simulink model "admire_sim_NDI"  (Simulink 9.1)
settings: Solver=ode4  StartTime=0.0  StopTime=500  FixedStep=dt  RelTol=1e-3  AbsTol=1e-6
InitFcn:
  | INIT_NDI
StartFcn:
  | tic
StopFcn:
  | toctime=toc;
  | fprintf('Actual Time = %g\nSim Time = %g\n',toctime,tout(end))
  | % Make plots
  | %admire_sim_plot
  | figure
  | plot3(yout(:,11),yout(:,10),-yout(:,12),'*-');grid
  | xlabel('East (m)');ylabel('North (m)');zlabel('Alt (m)')
  | view([0 0 1])
  | hold on
  | plot3(Ywpt,Xwpt,0*Xwpt,'r^-','MarkerSize',10)
  | axis equal
  | hold off
values from neighbouring files (symbols this model uses):
  a1 = (180*d2r)/(80^3)    (= 6.13592315154e-06)    [INIT_NDI.m]
  a2 = (24*d2r)/(80^3)    (= 8.18123086872e-07)    [INIT_NDI.m]
  Altcmd_t = [ 0    1   100 200  300  425  450  550  600  700  800  880  980]    [INIT_NDI.m]
  Altcmd_v = [20  20   20   1500 1500 1500 1500 3000 3000 4000 4000 6000 6000]    [INIT_NDI.m]
  bref = 10    [INIT_NDI.m]
  C1 = ((Iy-Iz)*Iz-Ixz^2)/GG    (= -0.958151081688)    [INIT_NDI.m]
  C2 = (Ix-Iy+Iz)*Ixz/GG    (= 0.0484690861804)    [INIT_NDI.m]
  C3 = Iz/GG    (= 4.77597824802e-05)    [INIT_NDI.m]
  C4 = Ixz/GG    (= 1.18217283367e-06)    [INIT_NDI.m]
  C5 = (Iz-Ix)/Iy    (= 0.987654320988)    [INIT_NDI.m]
  C6 = Ixz/Iy    (= 0.0308641975309)    [INIT_NDI.m]
  C7 = 1/Iy    (= 1.23456790123e-05)    [INIT_NDI.m]
  C8 = (Ix*(Ix-Iy)+Ixz^2)/GG    (= -0.592859676085)    [INIT_NDI.m]
  C9 = Ix/GG    (= 9.93025180281e-06)    [INIT_NDI.m]
  CAmethod = 6    [INIT_NDI.m]
  Canard_max = [25 25 25 15 15 15 15 15]*d2r    [INIT_NDI.m]
  Canard_min = [-55 -55 -25 -15 -15 -15 -15 -15]*d2r    [INIT_NDI.m]
  CB = CCV*Bbare    [INIT_NDI.m]
  CC = [C3 0 C4;0 C7 0;C4 0 C9]    [INIT_NDI.m]
  CCV = [CCV zeros(3,22)]    [INIT_NDI.m]
  cref = 5.2    [INIT_NDI.m]
  d2r = pi/180    (= 0.0174532925199)    [INIT_NDI.m]
  dt = 0.01    [INIT_NDI.m]
  DTY_max = 0.002    [INIT_NDI.m]
  DTY_min = -0.002    [INIT_NDI.m]
  DTZ_max = 0.002    [INIT_NDI.m]
  DTZ_min = -0.002    [INIT_NDI.m]
  du = [eye(7,7)*d2r eye(7,7)*(-d2r);zeros(20,14)]    [INIT_NDI.m]
  Elevon_max = [30 30 25 25 25 25 25 25]*d2r    [INIT_NDI.m]
  Elevon_min = [-30 -30 -30 -30 -30 -30 -30 -30]*d2r    [INIT_NDI.m]
  G = [ 0 1 0 ... (first row only)    [INIT_NDI.m]
  kcb = 2.5    [INIT_NDI.m]
  kfb = -0.4    [INIT_NDI.m]
  kib = 0.2    [INIT_NDI.m]
  kpb = 0.8    [INIT_NDI.m]
  LEF_max = [30 30 30 20 20 15 10 10]*d2r    [INIT_NDI.m]
  LEF_min = [-10 -10 -10 -10 -10 -10 -10 -10]*d2r    [INIT_NDI.m]
  LG_max = 1    [INIT_NDI.m]
  LG_min = 0    [INIT_NDI.m]
  LPmethod = 5    [INIT_NDI.m]    (also in LPwrap.m = 0)
  M_vec = [0 0.5 0.8 0.9 0.95 1.4 1.5 2.5]    [INIT_NDI.m]
  mass = 9100    [INIT_NDI.m]
  NumU = 16    [INIT_NDI.m]
  nwpt = 5    [INIT_NDI.m]
  PD_max = 10    [INIT_NDI.m]
  PD_min = -10    [INIT_NDI.m]
  PHIcmd_t = [0 1 1+dt 30 30+dt 60 60+dt 90 90+dt 120 120+dt 150 150+dt 180 180+dt 210 210+dt 240 240+dt 270 270+dt 300 300+dt 330 330+dt]    [INIT_NDI.m]
  PHIcmd_v = [0 0 15   15 -15   -15 0    0   30   30  -30    -30 0      0   45     45   0     0    -45   -45   0     0   -60   -60 0]    [INIT_NDI.m]
  Pmode = 3    [INIT_NDI.m]
  r2d = 180/pi    (= 57.2957795131)    [INIT_NDI.m]
  Rmode = 3    [INIT_NDI.m]
  Rudder_max = [30 30 25 20 15 15 15 10]*d2r    [INIT_NDI.m]
  Rudder_min = [-30 -30 -25 -20 -15 -15 -15 -10]*d2r    [INIT_NDI.m]
  Sref = 45    [INIT_NDI.m]
  TSS_max = 1    [INIT_NDI.m]
  TSS_min = 0    [INIT_NDI.m]
  UD_max = 10    [INIT_NDI.m]
  UD_min = -10    [INIT_NDI.m]
  Upref = [0 0 0 0 0 0 0 0 0 0 0 0 0 0 0 0]'    [INIT_NDI.m]
  Upref_split = [[0 0 30 -30 -30 30 0]*d2r*.4 0 0 0 0 0 0 0 0 0]'    [INIT_NDI.m]
  Urlim = [50*d2r ... (first row only)    [INIT_NDI.m]
  UseRL = 0    [INIT_NDI.m]
  Vcmd_t = [  0    1   100  200  300  425  450  550  600  700  800  880  980]    [INIT_NDI.m]
  Vcmd_v = Mcmd_v.*a    [INIT_NDI.m]
  VD_max = 10    [INIT_NDI.m]
  VD_min = -10    [INIT_NDI.m]
  WD_max = 10    [INIT_NDI.m]
  WD_min = -10    [INIT_NDI.m]
  Wp = W'*W    [INIT_NDI.m]
  Wpts = [0 1 2 3 4]    [INIT_NDI.m]
  x0 = [ max(eyp,zeros(n,1));max(-eyp,zeros(n,1));zeros(2*m,1)]    [LPwrap.m]
  Xwpt = [0 4000 4000 0 0]*8    [INIT_NDI.m]
  Ywpt = [0 0 4000 4000 0]*8    [INIT_NDI.m]
undefined symbols (not defined in the file or in its folder): Abare, Bbare, CGIwrap, dalpha_err, dalt_err, DAwrap, dbeta_err, ddc_bw, ddc_rate, ddei_bw, ddei_rate, ddey_bw, ddey_rate, ddle_bw, ddle_rate, ddr_bw, ddr_rate, DiscIntNeverNeededParam, dVt_err, LPwrap, rlimit_c, rlimit_ie, rlimit_le, rlimit_oe, rlimit_r, u0fcs, u0new, VJAwrap, x0bare, y0bare
libraries: simulink_extras x19, simulink x12
(part 1 of 4)
settings Model: Creator=ulrik  LastModifiedBy=Meng Chaoheng  ModifiedComment=nnt -- Mon Jun 05 13:08:11 2000 -- Version 3.42  ExtModeTrigMode=oneshot  ExtModeArmWhenConnect=off  ExtModeAutoUpdateStatusClock=off
settings Model: ModifiedHistory=|
  | nnt -- Mon Jun 05 13:08:11 2000 -- Version 3.42
  | 
  | 
  | nnt -- Mon Jun 05 11:01:33 2000 -- Version 3.41
  | 
  | 
  | nnt -- Mon Jun 05 10:57:40 2000 -- Version 3.40
  | 
  | 
  | nnt -- Mon Jun 05 10:56:46 2000 -- Version 3.39
  | 
  | 
  | hkg -- Thu Apr 13 16:38:30 2000 -- Version 3.38
  | Bug fix: all rate limiters were set with the canard parameters, now they get individual settings..
  | 
  | hkg -- Thu Apr 13 10:24:31 2000 -- Version 3.37
  | Inserted 3.0 version number in Level 1, changed month to April.
  | 
  | hkg -- Tue Apr 11 10:36:55 2000 -- Version 3.36
  | dtz re-connected
  | 
  | hkg -- Tue Apr 11 10:28:52 2000 -- Version 3.35
  | Changed the roll force saturation to +-80 N
  | 
  | hkg -- Tue Apr 11 09:23:02 2000 -- Version 3.34
  | All signal generators on Level 1 are now set to sine wave
  | 
  | hkg -- Mon Apr 10 15:03:16 2000 -- Version 3.33
  | New names for the RL_choice blocks
  | 
  | fosimadmin -- Mon Apr 10 13:44:14 2000 -- Version 3.32
  | Hkg actually. Nothing special
  | 
  | hkg -- Fri Apr 07 14:32:16 2000 -- Version 3.31
  | A few corrections to the names
  | 
  | hkg -- Fri Apr 07 14:16:55 2000 -- Version 3.30
  | Added unique names inside Saab and DASA rate limiters for left elevons, rudder and
  | leading-edge flaps.
  | hkg -- Fri Apr 07 14:04:35 2000 -- Version 3.29
  | Added unique names inside SAAB and DASA rate limiters for canard and right outer and
  | inner elevons.
  | hkg -- Thu Apr 06 17:23:24 2000 -- Version 3.28
  | Inserted unique names for rate limiters and multiport switches in the rate limiter selection blocks.
  | hkg -- Thu Apr 06 16:09:22 2000 -- Version 3.27
  | Disconnected dtz again. Chosen grt_adm5p3.tmf as template makefile. Code generation seems to work.
  | hyd -- Tue Mar 28 15:20:39 2000 -- Version 3.26
  | hyd -- Tue Mar 28 14:28:32 2000 -- Version 3.25
  | hyd -- Tue Mar 28 11:30:24 2000 -- Version 3.24
  | hyd -- Mon Mar 27 15:22:27 2000 -- Version 3.23
  | hyd -- Mon Mar 27 13:42:12 2000 -- Version 3.22
  | hyd -- Mon Mar 27 10:51:54 2000 -- Version 3.21
  | hyd -- Fri Mar 24 13:18:05 2000 -- Version 3.20
  | hyd -- Fri Mar 24 12:50:02 2000 -- Version 3.19
  | hyd -- Fri Mar 24 11:54:23 2000 -- Version 3.18
  | hyd -- Thu Mar 23 15:20:42 2000 -- Version 3.17
  | hyd -- Thu Mar 23 15:17:54 2000 -- Version 3.16
  | hyd -- Wed Mar 22 09:38:49 2000 -- Version 3.15
  | hyd -- Tue Mar 21 14:06:08 2000 -- Version 3.14
  | hyd -- Mon Mar 20 14:42:54 2000 -- Version 3.13
  | hyd -- Wed Mar 15 13:37:48 2000 -- Version 3.12
  | hyd -- Wed Mar 15 12:35:54 2000 -- Version 3.11
  | jnr -- Tue Mar 14 16:36:26 2000 -- Version 3.10
  | jnr -- Tue Mar 14 14:13:39 2000 -- Version 3.9
  | jnr -- Tue Mar 14 14:13:23 2000 -- Version 3.8
  | jnr -- Tue Mar 14 10:09:15 2000 -- Version 3.7
  | jnr -- Tue Mar 14 09:37:34 2000 -- Version 3.6
  | jnr -- Tue Mar 14 09:30:20 2000 -- Version 3.5
  | Add:
  | *proper stick gradients.
  | *correct gains for nz-control according to ke Hydn.
  | *what transition region between q-control and nz-control is proper??
  | fll -- Fri Mar 03 09:53:48 2000 -- Version 3.4
  | changed name of "dtx" to "dty" (horizontal nozzle deflection)
  | fll -- Thu Mar 02 12:51:23 2000 -- Version 3.3
  | Reducesed the number of integrators to one in the longitudinal controller.
  | fll -- Thu Mar 02 12:30:52 2000 -- Version 3.2
  | Moved the blending function in the Nz and q controller.
  | fll -- Thu Mar 02 10:50:25 2000 -- Version 3.1
  | Changed input blocks to "Signal generator"
  | fll -- Thu Mar 02 10:50:25 2000 -- Version 3.0
  | Version 3.0 is modified according to comments from users
settings SolverCC: AutoScaleAbsTol=off
settings DataIOCC: SignalLoggingName=sigsOut
settings OptimizationCC: BooleanDataType=off  ExpressionDepthLimit=2147483647
settings DebuggingCC: SaveWithParameterizedLinksMsg=none  CheckSSInitialOutputMsg=off  SignalResolutionControl=TryResolveAllWithWarning  MultiTaskDSMMsg=warning  MultiTaskCondExecSysMsg=none  FcnCallInpInsideContextMsg=warning  UnconnectedInputMsg=none  UnconnectedOutputMsg=none  UnconnectedLineMsg=none  StateNameClashWarn=warning
settings HardwareCC: TargetUnknown=on
settings RTWCC: TemplateMakefile=grt_adm5p3.tmf
settings GRTTargetCC: GeneratePreprocessorConditionals=Disable all
settings ConfigComp: CovSFcnEnable=off

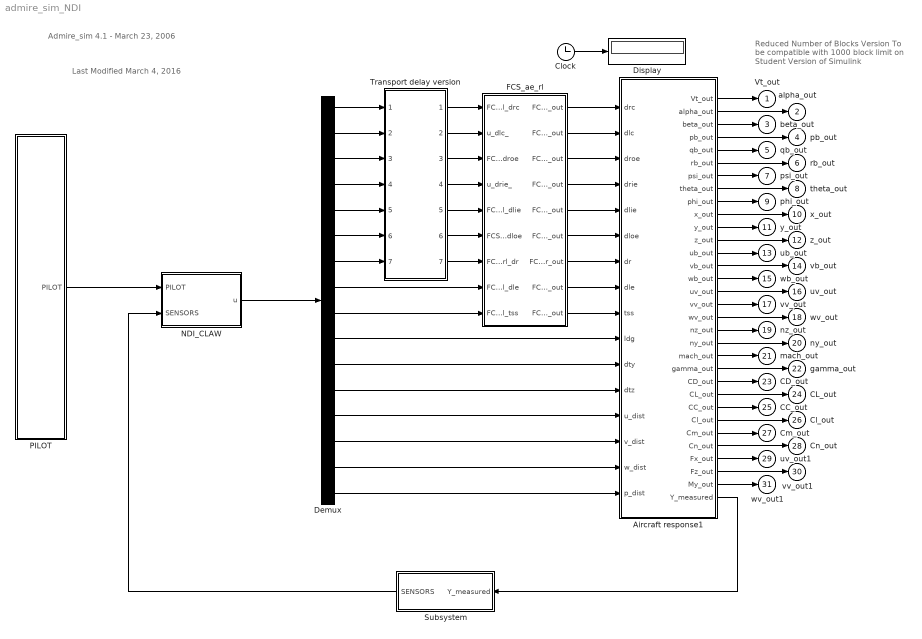
== system admire_sim_NDI ==
  note: Admire_sim 4.1 - March 23, 2006
  note: Reduced Number of Blocks Version
      | To be compatible with 1000 block limit
      | on Student Version of Simulink
  note: Last Modified
      | March 4, 2016
  Aircraft response1 : Subsystem
      mask Display: disp('Aircraft\nResponse')
  Clock : Clock
  Demux : Demux  Outputs=16
  Display : Display
  FCS_ae_rl : Subsystem
      mask Display: disp('Saturators\nRatelimiters\nand\nActuators')
  NDI_CLAW : Subsystem
  PILOT : Subsystem
  Subsystem : Subsystem
  Transport delay version : Subsystem
      mask Display: disp('Total\nComputer\nDelay\n\nTransport\ndelay\nversion')
  Vt_out : Outport  InitialOutput=0
  alpha_out : Outport  Port=2  InitialOutput=0
  beta_out : Outport  Port=3  InitialOutput=0
  pb_out : Outport  Port=4  InitialOutput=0
  qb_out : Outport  Port=5  InitialOutput=0
  rb_out : Outport  Port=6  InitialOutput=0
  psi_out : Outport  Port=7  InitialOutput=0
  theta_out : Outport  Port=8  InitialOutput=0
  phi_out : Outport  Port=9  InitialOutput=0
  x_out : Outport  Port=10  InitialOutput=0
  y_out : Outport  Port=11  InitialOutput=0
  z_out : Outport  Port=12  InitialOutput=0
  ub_out : Outport  Port=13  InitialOutput=0
  vb_out : Outport  Port=14  InitialOutput=0
  wb_out : Outport  Port=15  InitialOutput=0
  uv_out : Outport  Port=16  InitialOutput=0
  vv_out : Outport  Port=17  InitialOutput=0
  wv_out : Outport  Port=18  InitialOutput=0
  nz_out : Outport  Port=19  InitialOutput=0
  ny_out : Outport  Port=20  InitialOutput=0
  mach_out : Outport  Port=21  InitialOutput=0
  gamma_out : Outport  Port=22  InitialOutput=0
  CD_out : Outport  Port=23  InitialOutput=0
  CL_out : Outport  Port=24  InitialOutput=0
  CC_out : Outport  Port=25  InitialOutput=0
  Cl_out : Outport  Port=26  InitialOutput=0
  Cm_out : Outport  Port=27  InitialOutput=0
  Cn_out : Outport  Port=28  InitialOutput=0
  uv_out1 : Outport  Port=29  InitialOutput=0
  vv_out1 : Outport  Port=30  InitialOutput=0
  wv_out1 : Outport  Port=31  InitialOutput=0
  wires:
  Aircraft response1/1(Vt_out) -> Vt_out/1
  Aircraft response1/3(beta_out) -> beta_out/1
  Aircraft response1/5(qb_out) -> qb_out/1
  Aircraft response1/7(psi_out) -> psi_out/1
  Aircraft response1/9(phi_out) -> phi_out/1
  Aircraft response1/11(y_out) -> y_out/1
  Aircraft response1/13(ub_out) -> ub_out/1
  Aircraft response1/15(wb_out) -> wb_out/1
  Aircraft response1/19(nz_out) -> nz_out/1
  FCS_ae_rl/8(FCS_ae_rl_dle_out) -> Aircraft response1/8(dle)
  FCS_ae_rl/7(FCS_ae_rl_dr_out) -> Aircraft response1/7(dr)
  FCS_ae_rl/6(FCS_ae_rl_dloe_out) -> Aircraft response1/6(dloe)
  FCS_ae_rl/5(FCS_ae_rl_dlie_out) -> Aircraft response1/5(dlie)
  FCS_ae_rl/4(FCS_ae_rl_drie_out) -> Aircraft response1/4(drie)
  FCS_ae_rl/3(FCS_ae_rl_droe_out) -> Aircraft response1/3(droe)
  FCS_ae_rl/2(FCS_ae_rl_dlc_out) -> Aircraft response1/2(dlc)
  FCS_ae_rl/1(FCS_ae_rl_drc_out) -> Aircraft response1/1(drc)
  FCS_ae_rl/9(FCS_ae_rl_tss_out) -> Aircraft response1/9(tss)
  Transport delay version/1(FCS_ae_rl_del_drc_delayed) -> FCS_ae_rl/1(FCS_ae_rl_drc)
  Transport delay version/2(FCS_ae_rl_del_dlc_delayed) -> FCS_ae_rl/2(u_dlc_)
  Transport delay version/3(FCS_ae_rl_del_droe_delayed) -> FCS_ae_rl/3(FCS_ae_rl_droe)
  Transport delay version/4(FCS_ae_rl_del_drie_delayed) -> FCS_ae_rl/4(u_drie_)
  Transport delay version/5(FCS_ae_rl_del_dlie_delayed) -> FCS_ae_rl/5(FCS_ae_rl_dlie)
  Transport delay version/6(FCS_ae_rl_del_dloe_delayed) -> FCS_ae_rl/6(FCS_ae_rl_dloe)
  Transport delay version/7(FCS_ae_rl_del_dr_delayed) -> FCS_ae_rl/7(FCS_ae_rl_dr)
  Aircraft response1/17(vv_out) -> vv_out/1
  Aircraft response1/21(mach_out) -> mach_out/1
  Aircraft response1/23(CD_out) -> CD_out/1
  Aircraft response1/25(CC_out) -> CC_out/1
  Aircraft response1/27(Cm_out) -> Cm_out/1
  Aircraft response1/29(Fx_out) -> uv_out1/1
  Aircraft response1/31(My_out) -> wv_out1/1
  Aircraft response1/2(alpha_out) -> alpha_out/1
  Aircraft response1/22(gamma_out) -> gamma_out/1
  Aircraft response1/4(pb_out) -> pb_out/1
  Aircraft response1/6(rb_out) -> rb_out/1
  Aircraft response1/8(theta_out) -> theta_out/1
  Aircraft response1/10(x_out) -> x_out/1
  Aircraft response1/14(vb_out) -> vb_out/1
  Aircraft response1/16(uv_out) -> uv_out/1
  Aircraft response1/18(wv_out) -> wv_out/1
  Aircraft response1/20(ny_out) -> ny_out/1
  Aircraft response1/12(z_out) -> z_out/1
  Aircraft response1/24(CL_out) -> CL_out/1
  Aircraft response1/26(Cl_out) -> Cl_out/1
  Aircraft response1/28(Cn_out) -> Cn_out/1
  Aircraft response1/30(Fz_out) -> vv_out1/1
  Demux/1 -> Transport delay version/1(FCS_ae_rl_del_drc)
  Demux/2 -> Transport delay version/2(FCS_ae_rl_del_dlc)
  Demux/3 -> Transport delay version/3(FCS_ae_rl_del_droe)
  Demux/4 -> Transport delay version/4(FCS_ae_rl_del_drie)
  Demux/5 -> Transport delay version/5(FCS_ae_rl_del_dlie)
  Demux/6 -> Transport delay version/6(FCS_ae_rl_del_dloe)
  Demux/7 -> Transport delay version/7(FCS_ae_rl_del_dr)
  Demux/8 -> FCS_ae_rl/8(FCS_ae_rl_dle)
  Demux/9 -> FCS_ae_rl/9(FCS_ae_rl_tss)
  Demux/10 -> Aircraft response1/10(ldg)
  Demux/11 -> Aircraft response1/11(dty)
  Demux/13 -> Aircraft response1/13(u_dist)
  Demux/14 -> Aircraft response1/14(v_dist)
  Demux/15 -> Aircraft response1/15(w_dist)
  Demux/16 -> Aircraft response1/16(p_dist)
  Demux/12 -> Aircraft response1/12(dtz)
  Clock/1 -> Display/1
  PILOT/1(PILOT) -> NDI_CLAW/1(PILOT)
  NDI_CLAW/1(u) -> Demux/1
  Subsystem/1(SENSORS) -> NDI_CLAW/2(SENSORS)
  Aircraft response1/32(Y_measured) -> Subsystem/1(Y_measured)

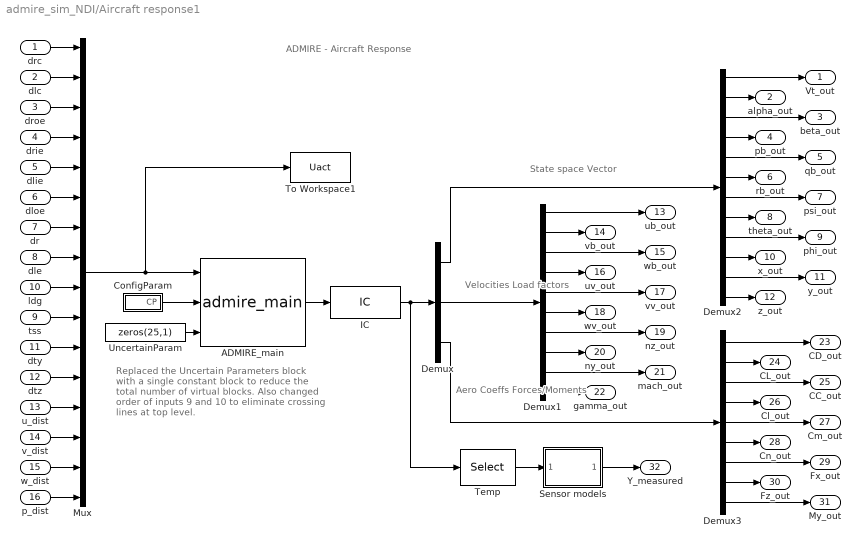
== system admire_sim_NDI/Aircraft response1 ==
  note: State space Vector
  note: Velocities
      | Load factors
  note: Aero Coeffs
      | Forces/Moments
  note: ADMIRE - Aircraft Response
  note: Replaced the Uncertain Parameters block
      | with a single constant block to reduce
      | the total number of virtual blocks.
      | Also changed order of inputs 9 and 10
      | to eliminate crossing lines at top level.
  drc : Inport
  dlc : Inport  Port=2
  droe : Inport  Port=3
  drie : Inport  Port=4
  dlie : Inport  Port=5
  dloe : Inport  Port=6
  dr : Inport  Port=7
  dle : Inport  Port=8
  tss : Inport  Port=9
  ldg : Inport  Port=10
  dty : Inport  Port=11
  dtz : Inport  Port=12
  u_dist : Inport  Port=13
  v_dist : Inport  Port=14
  w_dist : Inport  Port=15
  p_dist : Inport  Port=16
  ADMIRE_main : S-Function  FunctionName=admire_main  Parameters=x0bare dx0bare  SFunctionDeploymentMode=off  EnableBusSupport=off  mask(ADMIRE C-code block){}
      mask help:
      | Main block describing the ADMIRE.
      | To use HELP, start any Internet browser.
      mask Help:
      | The aircraft it self is a C-code file that calculates the dynamics of the structure and the air surrounding it.<br>
      | The simulation requires an initial vector of values called x0 containing the following variables.<br><br>
      | 
      | Vt_init     --     initial airspeed.                        [m/s]<br>
      | alpha_init --    initial angle of attack.             [rad]<br>
      | beta_init    --   initial angle of sideslip.            [rad]<br>
      | pb_init     --     initial roll angular rate.             [rad/s]<br>
      | qb_init     --     initial pitch angular rate.          [rad/s]<br>
      | rb_init       --    initial yaw angular rate.           [rad/s]<br>
      | psi_init      --    initial euler angles (azimuth)    [rad]<br>
      | theta_init   --   initial (elevation)                      [rad]<br>
      | phi_init      --   initial (bank)                             [rad]<br>
      | xv_init      --    initial x position in Fv                [m]<br>
      | yv_init        --  initial y                                     [m]<br>
      | zv_init       --   initial z                                     [m]<br>
      mask Display:
      | plot([18 12 3 2 2 8 11],[7 4 1 1 2 8 11])
      | plot([13 11 13 15 15 13],[12 11 16 17 13 12])
      | plot([15 17 20 23 30 17],[13 14 24 25 20 14])
      | plot([30 38 40 38 30],[19 31 32 22 19])
      | plot([38.5 41 36 22 41 43 36],[23 21 16 10 8 10 16])
      | plot([15 19 25 24 15],[7 9 9 8 7])
      | plot([8 11 13 14 9 8],[8 11 12 10 7 8])
      | plot([21 23],[9 10])
      | plot([30 31],[20 20.5])
  ConfigParam : Subsystem
  Demux : Demux  Outputs=[12 10 9]
  Demux1 : Demux  Outputs=10
  Demux2 : Demux  Outputs=12
  Demux3 : Demux  Outputs=9
  IC : InitialCondition  Value=y0bare(1:31)
  Mux : Mux  Inputs=16
  Sensor models : Subsystem
      mask Display: disp('Sensors')
  Temp : Selector  InputPortWidth=31  IndexOptions=Index vector (dialog)  Indices=[1:28]  OutputSizes=1
  To Workspace1 : ToWorkspace  VariableName=Uact  SampleTime=-1
  "UncertainParam " : Constant  Value=zeros(25,1)
  Vt_out : Outport
  alpha_out : Outport  Port=2
  beta_out : Outport  Port=3
  pb_out : Outport  Port=4
  qb_out : Outport  Port=5
  rb_out : Outport  Port=6
  psi_out : Outport  Port=7
  theta_out : Outport  Port=8
  phi_out : Outport  Port=9
  x_out : Outport  Port=10
  y_out : Outport  Port=11
  z_out : Outport  Port=12
  ub_out : Outport  Port=13
  vb_out : Outport  Port=14
  wb_out : Outport  Port=15
  uv_out : Outport  Port=16
  vv_out : Outport  Port=17
  wv_out : Outport  Port=18
  nz_out : Outport  Port=19
  ny_out : Outport  Port=20
  mach_out : Outport  Port=21
  gamma_out : Outport  Port=22
  CD_out : Outport  Port=23
  CL_out : Outport  Port=24
  CC_out : Outport  Port=25
  Cl_out : Outport  Port=26
  Cm_out : Outport  Port=27
  Cn_out : Outport  Port=28
  Fx_out : Outport  Port=29
  Fz_out : Outport  Port=30
  My_out : Outport  Port=31
  Y_measured : Outport  Port=32
  wires:
  Mux/1 -> ADMIRE_main/1, To Workspace1/1
  w_dist/1 -> Mux/15
  p_dist/1 -> Mux/16
  drc/1 -> Mux/1
  dlc/1 -> Mux/2
  droe/1 -> Mux/3
  drie/1 -> Mux/4
  dlie/1 -> Mux/5
  dloe/1 -> Mux/6
  dr/1 -> Mux/7
  dle/1 -> Mux/8
  ldg/1 -> Mux/9
  tss/1 -> Mux/10
  dty/1 -> Mux/11
  dtz/1 -> Mux/12
  u_dist/1 -> Mux/13
  v_dist/1 -> Mux/14
  Demux/2 -> Demux1/1
  Demux/1 -> Demux2/1
  Demux/3 -> Demux3/1
  Demux3/2 -> CL_out/1
  Demux3/4 -> Cl_out/1
  Demux3/6 -> Cn_out/1
  Demux3/8 -> Fz_out/1
  Demux3/1 -> CD_out/1
  Demux3/3 -> CC_out/1
  Demux3/5 -> Cm_out/1
  Demux3/7 -> Fx_out/1
  Demux3/9 -> My_out/1
  Demux2/2 -> alpha_out/1
  Demux2/4 -> pb_out/1
  Demux2/6 -> rb_out/1
  Demux2/8 -> theta_out/1
  Demux2/10 -> x_out/1
  Demux2/12 -> z_out/1
  Demux2/1 -> Vt_out/1
  Demux2/3 -> beta_out/1
  Demux2/5 -> qb_out/1
  Demux2/7 -> psi_out/1
  Demux2/9 -> phi_out/1
  Demux2/11 -> y_out/1
  Demux1/2 -> vb_out/1
  Demux1/4 -> uv_out/1
  Demux1/6 -> wv_out/1
  Demux1/8 -> ny_out/1
  Demux1/10 -> gamma_out/1
  Demux1/1 -> ub_out/1
  Demux1/3 -> wb_out/1
  Demux1/5 -> vv_out/1
  Demux1/7 -> nz_out/1
  Demux1/9 -> mach_out/1
  Sensor models/1(admire_sensed_out) -> Y_measured/1
  Temp/1 -> Sensor models/1(admire_out)
  ConfigParam/1(CP) -> ADMIRE_main/2
  "UncertainParam "/1 -> ADMIRE_main/3
  ADMIRE_main/1 -> IC/1
  IC/1 -> Demux/1, Temp/1

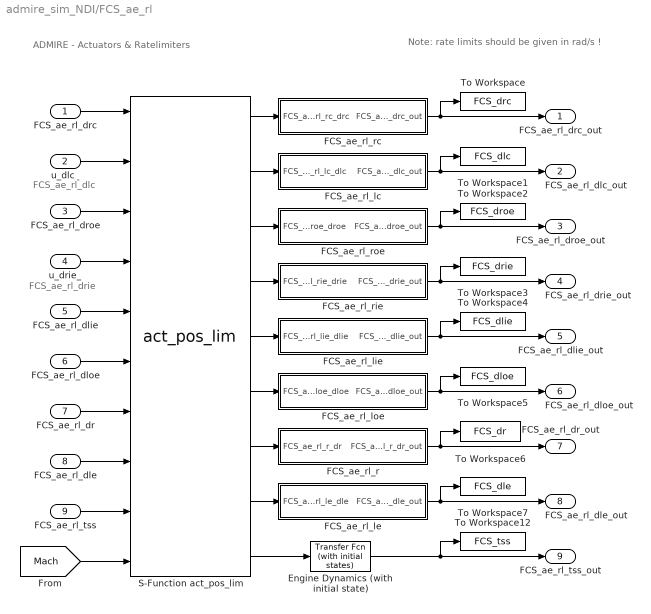
== system admire_sim_NDI/FCS_ae_rl ==
  note: Note: rate limits should be given
      | in rad/s !
  note: FCS_ae_rl_dlc
  note: FCS_ae_rl_drie
  note: ADMIRE - Actuators & Ratelimiters
  FCS_ae_rl_drc : Inport
  u_dlc_ : Inport  Port=2
  FCS_ae_rl_droe : Inport  Port=3
  u_drie_ : Inport  Port=4
  FCS_ae_rl_dlie : Inport  Port=5
  FCS_ae_rl_dloe : Inport  Port=6
  FCS_ae_rl_dr : Inport  Port=7
  FCS_ae_rl_dle : Inport  Port=8
  FCS_ae_rl_tss : Inport  Port=9
  Engine Dynamics (with initial state) : simulink_extras/Additional Linear/Transfer Fcn (with initial states)  N=[1]  D="[2  1]"  X0=x0(9)
  FCS_ae_rl_lc : Subsystem
      mask Display: disp(' Ratelimiter and Dynamics\nServo: lc')
  FCS_ae_rl_le : Subsystem
      mask Display: disp(' Ratelimiter and Dynamics\nServo: le')
  FCS_ae_rl_lie : Subsystem
      mask Display: disp(' Ratelimiter and Dynamics\nServo: lie')
  FCS_ae_rl_loe : Subsystem
      mask Display: disp(' Ratelimiter and Dynamics\nServo: loe')
  FCS_ae_rl_r : Subsystem
      mask Display: disp(' Ratelimiter and Dynamics\nServo: r')
  FCS_ae_rl_rc : Subsystem
      mask Display: disp(' Ratelimiter and Dynamics\nServo: rc')
  FCS_ae_rl_rie : Subsystem
      mask Display: disp(' Ratelimiter and Dynamics\nServo: rie')
  FCS_ae_rl_roe : Subsystem
      mask Display: disp(' Ratelimiter and Dynamics\nServo: roe')
  S-Function act_pos_lim : S-Function  FunctionName=act_pos_lim  SFunctionDeploymentMode=off  EnableBusSupport=off
      mask Display:
      | plot([-30 30],[-30 30])
      | plot([0 0],[-30 30])
      | plot([-50 50],[0 0])
      | plot([30 50],[30 30])
      | plot([-50 -30],[-30 -30])
      | plot([-5 0],[25 30])
      | plot([5 0],[25 30])
      | plot([45 50],[3 0])
      | plot([45 50],[-3 0])
      | text(-21,26,'out')
      | text(30,-2,'in')
  To Workspace : ToWorkspace  VariableName=FCS_drc  SampleTime=-1
  To Workspace1 : ToWorkspace  VariableName=FCS_dlc  SampleTime=-1
  To Workspace12 : ToWorkspace  VariableName=FCS_tss  SampleTime=-1
  To Workspace2 : ToWorkspace  VariableName=FCS_droe  SampleTime=-1
  To Workspace3 : ToWorkspace  VariableName=FCS_drie  SampleTime=-1
  To Workspace4 : ToWorkspace  VariableName=FCS_dlie  SampleTime=-1
  To Workspace5 : ToWorkspace  VariableName=FCS_dloe  SampleTime=-1
  To Workspace6 : ToWorkspace  VariableName=FCS_dr  SampleTime=-1
  To Workspace7 : ToWorkspace  VariableName=FCS_dle  SampleTime=-1
  FCS_ae_rl_drc_out : Outport
  FCS_ae_rl_dlc_out : Outport  Port=2
  FCS_ae_rl_droe_out : Outport  Port=3
  FCS_ae_rl_drie_out : Outport  Port=4
  FCS_ae_rl_dlie_out : Outport  Port=5
  FCS_ae_rl_dloe_out : Outport  Port=6
  FCS_ae_rl_dr_out : Outport  Port=7
  FCS_ae_rl_dle_out : Outport  Port=8
  FCS_ae_rl_tss_out : Outport  Port=9
  wires:
  S-Function act_pos_lim/2 -> FCS_ae_rl_lc/1(FCS_ae_rl_lc_dlc)
  S-Function act_pos_lim/3 -> FCS_ae_rl_roe/1(FCS_ae_rl_roe_droe)
  S-Function act_pos_lim/5 -> FCS_ae_rl_lie/1(FCS_ae_rl_lie_dlie)
  S-Function act_pos_lim/6 -> FCS_ae_rl_loe/1(FCS_ae_rl_loe_dloe)
  S-Function act_pos_lim/7 -> FCS_ae_rl_r/1(FCS_ae_rl_r_dr)
  S-Function act_pos_lim/8 -> FCS_ae_rl_le/1(FCS_ae_rl_le_dle)
  S-Function act_pos_lim/9 -> Engine Dynamics (with initial state)/1
  S-Function act_pos_lim/1 -> FCS_ae_rl_rc/1(FCS_ae_rl_rc_drc)
  S-Function act_pos_lim/4 -> FCS_ae_rl_rie/1(FCS_ae_rl_rie_drie)
  [Mach] -> S-Function act_pos_lim/10
  u_dlc_/1 -> S-Function act_pos_lim/2
  FCS_ae_rl_drc/1 -> S-Function act_pos_lim/1
  FCS_ae_rl_droe/1 -> S-Function act_pos_lim/3
  FCS_ae_rl_dlie/1 -> S-Function act_pos_lim/5
  FCS_ae_rl_dloe/1 -> S-Function act_pos_lim/6
  FCS_ae_rl_dr/1 -> S-Function act_pos_lim/7
  u_drie_/1 -> S-Function act_pos_lim/4
  FCS_ae_rl_dle/1 -> S-Function act_pos_lim/8
  FCS_ae_rl_tss/1 -> S-Function act_pos_lim/9
  FCS_ae_rl_rc/1(FCS_ae_rl_rc_drc_out) -> To Workspace/1, FCS_ae_rl_drc_out/1
  FCS_ae_rl_lc/1(FCS_ae_rl_lc_dlc_out) -> To Workspace1/1, FCS_ae_rl_dlc_out/1
  FCS_ae_rl_le/1(FCS_ae_rl_le_dle_out) -> To Workspace7/1, FCS_ae_rl_dle_out/1
  FCS_ae_rl_r/1(FCS_ae_rl_r_dr_out) -> To Workspace6/1, FCS_ae_rl_dr_out/1
  FCS_ae_rl_loe/1(FCS_ae_rl_loe_dloe_out) -> To Workspace5/1, FCS_ae_rl_dloe_out/1
  FCS_ae_rl_lie/1(FCS_ae_rl_lie_dlie_out) -> To Workspace4/1, FCS_ae_rl_dlie_out/1
  FCS_ae_rl_roe/1(FCS_ae_rl_roe_droe_out) -> To Workspace2/1, FCS_ae_rl_droe_out/1
  FCS_ae_rl_rie/1(FCS_ae_rl_rie_drie_out) -> To Workspace3/1, FCS_ae_rl_drie_out/1
  Engine Dynamics (with initial state)/1 -> To Workspace12/1, FCS_ae_rl_tss_out/1

== system admire_sim_NDI/NDI_CLAW ==
  PILOT : Inport
  SENSORS : Inport  Port=2
  DynamicInversionControl : Subsystem
  INPUT : Subsystem
  MissionManager : Subsystem
  PILOT_Mod : Subsystem
  Rate Transition : RateTransition  OutPortSampleTime=dt
  u : Outport
  wires:
  INPUT/1(INPUT) -> DynamicInversionControl/1(INPUT), MissionManager/1(INPUT)
  PILOT_Mod/1(PILOT) -> INPUT/1(PILOT)
  Rate Transition/1 -> INPUT/2(TIME_DELAY)
  PILOT/1 -> PILOT_Mod/1(In1)
  SENSORS/1 -> Rate Transition/1
  DynamicInversionControl/1(DI_Cmds) -> u/1
  MissionManager/1(MM) -> DynamicInversionControl/2(MM)

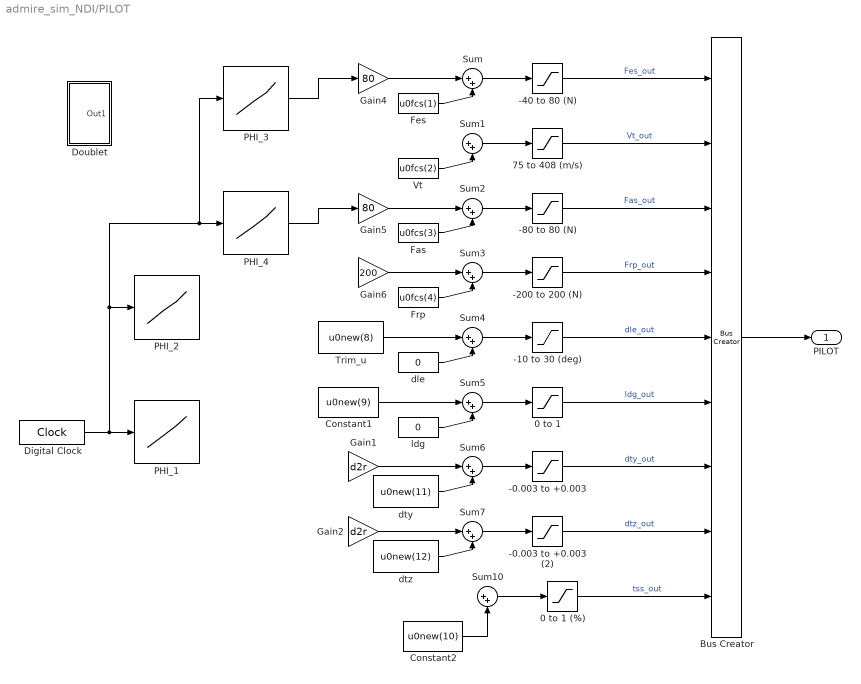
== system admire_sim_NDI/PILOT ==
  -0.003 to +0.003 : Saturate  UpperLimit=0.003  LowerLimit=-0.003
  -0.003 to +0.003 (2) : Saturate  UpperLimit=0.003  LowerLimit=-0.003
  -10 to 30 (deg) : Saturate  UpperLimit=30  LowerLimit=-10
  -200 to 200 (N) : Saturate  UpperLimit=200  LowerLimit=-200
  -40 to 80 (N) : Saturate  UpperLimit=80  LowerLimit=-40
  -80 to 80 (N) : Saturate  UpperLimit=80  LowerLimit=-80
  0 to 1 : Saturate  UpperLimit=1  LowerLimit=0
  0 to 1 (%) : Saturate  UpperLimit=1  LowerLimit=0
  75 to 408 (m/s) : Saturate  UpperLimit=408  LowerLimit=75
  Bus Creator : BusCreator  Inputs=9
  Constant1 : Constant  Value=u0new(9)
  Constant2 : Constant  Value=u0new(10)
  Digital Clock : DigitalClock  SampleTime=dt
  Doublet : Subsystem
  Fas : Constant  Value=u0fcs(3)
  Fes : Constant  Value=u0fcs(1)
  Frp : Constant  Value=u0fcs(4)
  Gain1 : Gain  Gain=d2r
  Gain2 : Gain  Gain=d2r
  Gain4 : Gain  Gain=80
  Gain5 : Gain  Gain=80
  Gain6 : Gain  Gain=200
  PHI_1 : Lookup  InputValues=[0 1 1+dt 4 10 10+dt 14 20 20+dt 24]  Table=[0 0 0.5 0 0 -1 0 0 0.5 0]*.45  LookUpMeth=Interpolation-Use End Values
  PHI_2 : Lookup  InputValues=[0 1 1+dt 4 10 10+dt 14 20 20+dt 24]  Table=[0 0 1 1 1 1 1 1 1 0]*.45  LookUpMeth=Interpolation-Use End Values
  PHI_3 : Lookup  InputValues=[0 50 50+dt 52 52+dt 70]  Table=[0 0 1 1 0.68 0.68]*60/80  LookUpMeth=Interpolation-Use End Values
  PHI_4 : Lookup  InputValues=[0 51 51+dt 54.5 54.5+dt 70]  Table=[0 0 1 1 0 0]*69/80  LookUpMeth=Interpolation-Use End Values
  Sum{,1..7,10} (9 alike) : Sum  Inputs=|++
  Trim_u : Constant  Value=u0new(8)
  Vt : Constant  Value=u0fcs(2)
  dle : Constant  Value=0
  dty : Constant  Value=u0new(11)
  dtz : Constant  Value=u0new(12)
  ldg : Constant  Value=0
  PILOT : Outport
  wires:
  Sum/1 -> -40 to 80 (N)/1
  Sum1/1 -> 75 to 408 (m/s)/1
  Sum2/1 -> -80 to 80 (N)/1
  Sum3/1 -> -200 to 200 (N)/1
  Sum4/1 -> -10 to 30 (deg)/1
  Sum5/1 -> 0 to 1/1
  Sum6/1 -> -0.003 to +0.003/1
  Sum7/1 -> -0.003 to +0.003 (2)/1
  Fes/1 -> Sum/2
  Vt/1 -> Sum1/2
  Fas/1 -> Sum2/2
  Frp/1 -> Sum3/2
  dle/1 -> Sum4/2
  ldg/1 -> Sum5/2
  dty/1 -> Sum6/2
  dtz/1 -> Sum7/2
  Gain1/1 -> Sum6/1
  Gain2/1 -> Sum7/1
  -40 to 80 (N)/1 -> Bus Creator/1  "Fes_out"
  75 to 408 (m/s)/1 -> Bus Creator/2  "Vt_out"
  -80 to 80 (N)/1 -> Bus Creator/3  "Fas_out"
  -200 to 200 (N)/1 -> Bus Creator/4  "Frp_out"
  -10 to 30 (deg)/1 -> Bus Creator/5  "dle_out"
  0 to 1/1 -> Bus Creator/6  "ldg_out"
  -0.003 to +0.003/1 -> Bus Creator/7  "dty_out"
  -0.003 to +0.003 (2)/1 -> Bus Creator/8  "dtz_out"
  Bus Creator/1 -> PILOT/1
  Constant1/1 -> Sum5/1
  Gain4/1 -> Sum/1
  Gain5/1 -> Sum2/1
  Gain6/1 -> Sum3/1
  Trim_u/1 -> Sum4/1
  Digital Clock/1 -> PHI_1/1, PHI_2/1, PHI_4/1, PHI_3/1
  Constant2/1 -> Sum10/2
  Sum10/1 -> 0 to 1 (%)/1
  0 to 1 (%)/1 -> Bus Creator/9  "tss_out"
  PHI_4/1 -> Gain5/1
  PHI_3/1 -> Gain4/1

== system admire_sim_NDI/Subsystem ==
  note: Modify heading angle to be between 0 and 360 deg (2*pi radians)
      | to better emulate a heading sensor
  Y_measured : Inport
  Assignment : Assignment  IndexOptions=Index vector (dialog)  Indices=7  OutputSizes=1
  Constant : Constant  Value=2*pi
  Math Function : Math  Operator=mod  SaturateOnIntegerOverflow=on
  Selector : Selector  InputPortWidth=28  IndexOptions=Index vector (dialog)  Indices=[7]  OutputSizes=1
  SENSORS : Outport
  wires:
  Y_measured/1 -> Selector/1, Assignment/1
  Assignment/1 -> SENSORS/1
  Constant/1 -> Math Function/2
  Selector/1 -> Math Function/1
  Math Function/1 -> Assignment/2

== system admire_sim_NDI/Transport delay version ==
  note: Level V
  FCS_ae_rl_del_drc : Inport
  FCS_ae_rl_del_dlc : Inport  Port=2
  FCS_ae_rl_del_droe : Inport  Port=3
  FCS_ae_rl_del_drie : Inport  Port=4
  FCS_ae_rl_del_dlie : Inport  Port=5
  FCS_ae_rl_del_dloe : Inport  Port=6
  FCS_ae_rl_del_dr : Inport  Port=7
  "20 ms Transport Delay, initial input from  u0new 1" : TransportDelay  DelayTime=0.02  InitialOutput=u0new(1)  BufferSize=100
  "20 ms Transport Delay, initial input from  u0new 2" : TransportDelay  DelayTime=0.02  InitialOutput=u0new(2)  BufferSize=100
  "20 ms Transport Delay, initial input from  u0new 3" : TransportDelay  DelayTime=0.02  InitialOutput=u0new(3)  BufferSize=100
  "20 ms Transport Delay, initial input from  u0new 4" : TransportDelay  DelayTime=0.02  InitialOutput=u0new(4)  BufferSize=100
  "20 ms Transport Delay, initial input from  u0new 5" : TransportDelay  DelayTime=0.02  InitialOutput=u0new(5)  BufferSize=100
  "20 ms Transport Delay, initial input from  u0new 6" : TransportDelay  DelayTime=0.02  InitialOutput=u0new(6)  BufferSize=100
  "20 ms Transport Delay, initial input from  u0new 7" : TransportDelay  DelayTime=0.02  InitialOutput=u0new(7)  BufferSize=100
  FCS_ae_rl_del_drc_delayed : Outport
  FCS_ae_rl_del_dlc_delayed : Outport  Port=2
  FCS_ae_rl_del_droe_delayed : Outport  Port=3
  FCS_ae_rl_del_drie_delayed : Outport  Port=4
  FCS_ae_rl_del_dlie_delayed : Outport  Port=5
  FCS_ae_rl_del_dloe_delayed : Outport  Port=6
  FCS_ae_rl_del_dr_delayed : Outport  Port=7
  wires:
  FCS_ae_rl_del_dloe/1 -> "20 ms Transport Delay, initial input from  u0new 6"/1
  "20 ms Transport Delay, initial input from  u0new 5"/1 -> FCS_ae_rl_del_dlie_delayed/1
  FCS_ae_rl_del_dlie/1 -> "20 ms Transport Delay, initial input from  u0new 5"/1
  FCS_ae_rl_del_drie/1 -> "20 ms Transport Delay, initial input from  u0new 4"/1
  "20 ms Transport Delay, initial input from  u0new 3"/1 -> FCS_ae_rl_del_droe_delayed/1
  FCS_ae_rl_del_droe/1 -> "20 ms Transport Delay, initial input from  u0new 3"/1
  "20 ms Transport Delay, initial input from  u0new 7"/1 -> FCS_ae_rl_del_dr_delayed/1
  "20 ms Transport Delay, initial input from  u0new 1"/1 -> FCS_ae_rl_del_drc_delayed/1
  FCS_ae_rl_del_drc/1 -> "20 ms Transport Delay, initial input from  u0new 1"/1
  "20 ms Transport Delay, initial input from  u0new 2"/1 -> FCS_ae_rl_del_dlc_delayed/1
  FCS_ae_rl_del_dlc/1 -> "20 ms Transport Delay, initial input from  u0new 2"/1
  "20 ms Transport Delay, initial input from  u0new 4"/1 -> FCS_ae_rl_del_drie_delayed/1
  "20 ms Transport Delay, initial input from  u0new 6"/1 -> FCS_ae_rl_del_dloe_delayed/1
  FCS_ae_rl_del_dr/1 -> "20 ms Transport Delay, initial input from  u0new 7"/1

== system admire_sim_NDI/Aircraft response1/ConfigParam ==
  note: Level II
  "Ix " : Constant  Value=21000
  "Ixz " : Constant  Value=2500
  "Iy " : Constant  Value=81000
  "Iz " : Constant  Value=101000
  Mux : Mux  Inputs=8
  "mass " : Constant  Value=9100
  "xcg " : Constant  Value=0*5.20
  "ycg " : Constant  Value=0
  "zcg " : Constant  Value=-0.15
  CP : Outport  InitialOutput=0
  wires:
  "mass "/1 -> Mux/1
  "xcg "/1 -> Mux/2
  "ycg "/1 -> Mux/3
  "zcg "/1 -> Mux/4
  "Ix "/1 -> Mux/5
  "Iy "/1 -> Mux/6
  "Iz "/1 -> Mux/7
  "Ixz "/1 -> Mux/8
  Mux/1 -> CP/1

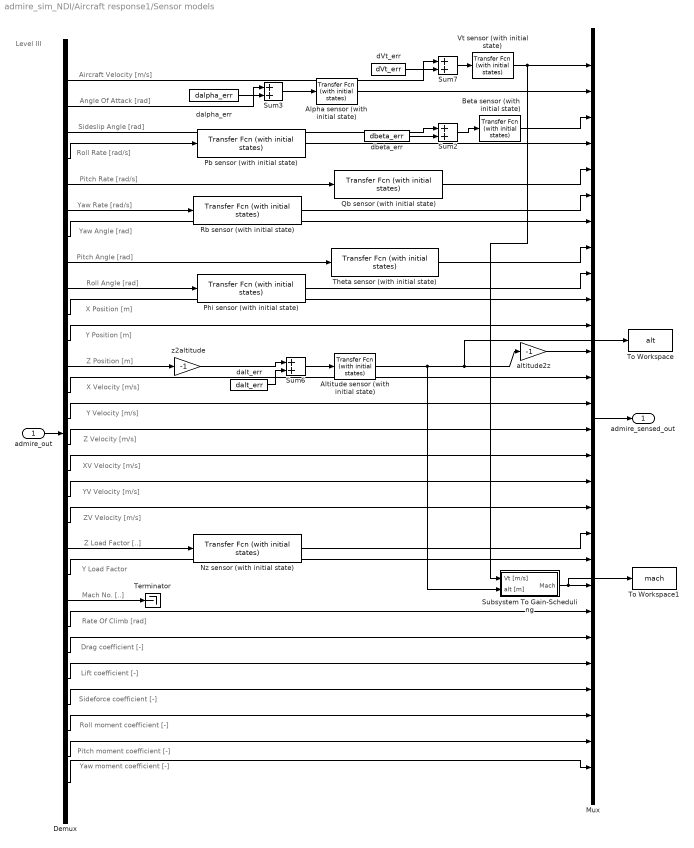
== system admire_sim_NDI/Aircraft response1/Sensor models ==
  note: Aircraft Velocity [m/s]
  note: Angle Of Attack [rad]
  note: Sideslip Angle [rad]
  note: Roll Rate [rad/s]
  note: Pitch Rate [rad/s]
  note: Yaw Rate [rad/s]
  note: Yaw Angle [rad]
  note: Pitch Angle [rad]
  note: Roll Angle [rad]
  note: X Position [m]
  note: Y Position [m]
  note: Z Position [m]
  note: X Velocity [m/s]
  note: Y Velocity [m/s]
  note: Z Velocity [m/s]
  note: ZV Velocity [m/s]
  note: YV Velocity [m/s]
  note: XV Velocity [m/s]
  note: Z Load Factor [..]
  note: Y Load Factor
  note: Mach No. [..]
  note: Rate Of Climb [rad]
  note: Drag coefficient [-]
  note: Lift coefficient [-]
  note: Sideforce coefficient [-]
  note: Roll moment coefficient [-]
  note: Pitch moment coefficient [-]
  note: Yaw moment coefficient [-]
  note: Level III
  admire_out : Inport
  Alpha sensor (with initial state) : simulink_extras/Additional Linear/Transfer Fcn (with initial states)  N=[1]  D="[0.02  1]"  X0=x0(23)
  Altitude sensor (with initial state) : simulink_extras/Additional Linear/Transfer Fcn (with initial states)  N=[1]  D="[0.02  1]"  X0=x0(35)
  Beta sensor (with initial state) : simulink_extras/Additional Linear/Transfer Fcn (with initial states)  N=[1]  D="[0.02  1]"  X0=x0(24)
  Demux : Demux  Outputs=28
  Mux : Mux  Inputs=28
  Nz sensor (with initial state) : simulink_extras/Additional Linear/Transfer Fcn (with initial states)  N=[0.0001903 0.005346 1]  D=[0.0004942 0.03082 1]  X0=[x0(36) x0(37)]
  Pb sensor (with initial state) : simulink_extras/Additional Linear/Transfer Fcn (with initial states)  N=[0.0001903 0.005346 1]  D=[0.0004942 0.03082 1]  X0=[x0(25) x0(26)]
  Phi sensor (with initial state) : simulink_extras/Additional Linear/Transfer Fcn (with initial states)  N=[1]  D=[0.00104 0.0323 1]  X0=[x0(33) x0(34)]
  Qb sensor (with initial state) : simulink_extras/Additional Linear/Transfer Fcn (with initial states)  N=[0.0001903 0.005346 1]  D=[0.0004942 0.03082 1]  X0=[x0(27) x0(28)]
  Rb sensor (with initial state) : simulink_extras/Additional Linear/Transfer Fcn (with initial states)  N=[0.0001903 0.005346 1]  D=[0.0004942 0.03082 1]  X0=[x0(29) x0(30)]
  Subsystem To Gain-Scheduling : Subsystem
  Sum{2..3,6..7} (4 alike) : Sum  SaturateOnIntegerOverflow=on  InputSameDT=on  OutDataTypeStr=Inherit: Same as first input
  Terminator : Terminator
  Theta sensor (with initial state) : simulink_extras/Additional Linear/Transfer Fcn (with initial states)  N=[1]  D=[0.00104 0.0323 1]  X0=[x0(31) x0(32)]
  To Workspace : ToWorkspace  VariableName=alt  SampleTime=-1
  To Workspace1 : ToWorkspace  VariableName=mach  SampleTime=-1
  Vt sensor (with initial state) : simulink_extras/Additional Linear/Transfer Fcn (with initial states)  N=[1]  D="[0.02  1]"  X0=x0(22)
  altitude2z : Gain  Gain=-1  OutDataTypeStr=Inherit: Same as input  ParamDataTypeStr=Inherit: Same as input
  dVt_err : Constant  Value=dVt_err
  dalpha_err : Constant  Value=dalpha_err
  dalt_err : Constant  Value=dalt_err
  dbeta_err : Constant  Value=dbeta_err
  z2altitude : Gain  Gain=-1  OutDataTypeStr=Inherit: Same as input  ParamDataTypeStr=Inherit: Same as input
  admire_sensed_out : Outport
  wires:
  Demux/24 -> Mux/24
  Demux/25 -> Mux/25
  Demux/26 -> Mux/26
  Demux/27 -> Mux/27
  Demux/28 -> Mux/28
  admire_out/1 -> Demux/1
  Qb sensor (with initial state)/1 -> Mux/5
  Demux/11 -> Mux/11
  Demux/13 -> Mux/13
  Demux/14 -> Mux/14
  Demux/5 -> Qb sensor (with initial state)/1
  Demux/4 -> Pb sensor (with initial state)/1
  Pb sensor (with initial state)/1 -> Mux/4
  Alpha sensor (with initial state)/1 -> Mux/2
  Demux/6 -> Rb sensor (with initial state)/1
  Rb sensor (with initial state)/1 -> Mux/6
  Demux/8 -> Theta sensor (with initial state)/1
  Theta sensor (with initial state)/1 -> Mux/8
  Demux/15 -> Mux/15
  Demux/16 -> Mux/16
  Demux/17 -> Mux/17
  Demux/18 -> Mux/18
  Demux/20 -> Mux/20
  Demux/22 -> Mux/22
  Demux/23 -> Mux/23
  Demux/21 -> Terminator/1
  dalpha_err/1 -> Sum3/2
  Demux/2 -> Sum3/1
  Sum3/1 -> Alpha sensor (with initial state)/1
  dbeta_err/1 -> Sum2/2
  Demux/3 -> Sum2/1
  Mux/1 -> admire_sensed_out/1
  Sum7/1 -> Vt sensor (with initial state)/1
  dVt_err/1 -> Sum7/2
  Demux/1 -> Sum7/1
  Vt sensor (with initial state)/1 -> Mux/1, Subsystem To Gain-Scheduling/1(Vt [m/s])
  Demux/9 -> Phi sensor (with initial state)/1
  Phi sensor (with initial state)/1 -> Mux/9
  Demux/7 -> Mux/7
  dalt_err/1 -> Sum6/2
  Sum6/1 -> Altitude sensor (with initial state)/1
  Demux/12 -> z2altitude/1
  z2altitude/1 -> Sum6/1
  Nz sensor (with initial state)/1 -> Mux/19
  Sum2/1 -> Beta sensor (with initial state)/1
  Beta sensor (with initial state)/1 -> Mux/3
  Demux/10 -> Mux/10
  Demux/19 -> Nz sensor (with initial state)/1
  altitude2z/1 -> Mux/12
  Altitude sensor (with initial state)/1 -> Subsystem To Gain-Scheduling/2(alt [m]), altitude2z/1, To Workspace/1
  Subsystem To Gain-Scheduling/1(Mach) -> Mux/21, To Workspace1/1

== system admire_sim_NDI/FCS_ae_rl/FCS_ae_rl_lc ==
  note: Level V
  FCS_ae_rl_lc_dlc : Inport
  RL2 : RateLimiter  RisingSlewLimit=rlimit_c+ddc_rate  FallingSlewLimit=-rlimit_c-ddc_rate
  dlc_actuator (with initial state) : simulink_extras/Additional Linear/Transfer Fcn (with initial states)  N=[1]  D="[0.05+ddc_bw  1]"  X0=x0(2)
  dlc_l : ToWorkspace  VariableName=dlc_l
  dlc_r : ToWorkspace  VariableName=dlc_r
  FCS_ae_rl_lc_dlc_out : Outport  InitialOutput=0
  wires:
  FCS_ae_rl_lc_dlc/1 -> dlc_l/1, RL2/1
  dlc_actuator (with initial state)/1 -> FCS_ae_rl_lc_dlc_out/1
  RL2/1 -> dlc_r/1, dlc_actuator (with initial state)/1

== system admire_sim_NDI/FCS_ae_rl/FCS_ae_rl_le ==
  note: Level V
  FCS_ae_rl_le_dle : Inport
  RL2 : RateLimiter  RisingSlewLimit=rlimit_le+ddle_rate  FallingSlewLimit=-rlimit_le-ddle_rate
  dle_actuator (with initial state) : simulink_extras/Additional Linear/Transfer Fcn (with initial states)  N=[1]  D="[0.05+ddle_bw  1]"  X0=x0(8)
  dle_l : ToWorkspace  VariableName=dle_l
  dle_r : ToWorkspace  VariableName=dle_r
  FCS_ae_rl_le_dle_out : Outport  InitialOutput=0
  wires:
  FCS_ae_rl_le_dle/1 -> dle_l/1, RL2/1
  dle_actuator (with initial state)/1 -> FCS_ae_rl_le_dle_out/1
  RL2/1 -> dle_r/1, dle_actuator (with initial state)/1

== system admire_sim_NDI/FCS_ae_rl/FCS_ae_rl_lie ==
  note: Level V
  FCS_ae_rl_lie_dlie : Inport
  RL2 : RateLimiter  RisingSlewLimit=rlimit_ie+ddei_rate  FallingSlewLimit=-rlimit_ie-ddei_rate
  dlie_actuator (with initial state) : simulink_extras/Additional Linear/Transfer Fcn (with initial states)  N=[1]  D="[0.05+ddei_bw  1]"  X0=x0(5)
  dlie_l : ToWorkspace  VariableName=dlie_l
  dlie_r : ToWorkspace  VariableName=dlie_r
  FCS_ae_rl_lie_dlie_out : Outport  InitialOutput=0
  wires:
  dlie_actuator (with initial state)/1 -> FCS_ae_rl_lie_dlie_out/1
  FCS_ae_rl_lie_dlie/1 -> dlie_l/1, RL2/1
  RL2/1 -> dlie_actuator (with initial state)/1, dlie_r/1

== system admire_sim_NDI/FCS_ae_rl/FCS_ae_rl_loe ==
  note: Level V
  FCS_ae_rl_loe_dloe : Inport
  RL2 : RateLimiter  RisingSlewLimit=rlimit_oe+ddey_rate  FallingSlewLimit=-rlimit_oe-ddey_rate
  dloe_actuator (with initial state) : simulink_extras/Additional Linear/Transfer Fcn (with initial states)  N=[1]  D="[0.05+ddey_bw  1]"  X0=x0(6)
  dloe_l : ToWorkspace  VariableName=dloe_l
  dloe_r : ToWorkspace  VariableName=dloe_r
  FCS_ae_rl_loe_dloe_out : Outport  InitialOutput=0
  wires:
  FCS_ae_rl_loe_dloe/1 -> dloe_l/1, RL2/1
  dloe_actuator (with initial state)/1 -> FCS_ae_rl_loe_dloe_out/1
  RL2/1 -> dloe_r/1, dloe_actuator (with initial state)/1

== system admire_sim_NDI/FCS_ae_rl/FCS_ae_rl_r ==
  note: Level V
  FCS_ae_rl_r_dr : Inport
  RL2 : RateLimiter  RisingSlewLimit=rlimit_r+ddr_rate  FallingSlewLimit=-rlimit_r-ddr_rate
  dr_actuator (with initial state) : simulink_extras/Additional Linear/Transfer Fcn (with initial states)  N=[1]  D="[0.05+ddr_bw  1]"  X0=x0(7)
  dr_l : ToWorkspace  VariableName=dr_l
  dr_r : ToWorkspace  VariableName=dr_r
  FCS_ae_rl_r_dr_out : Outport  InitialOutput=0
  wires:
  dr_actuator (with initial state)/1 -> FCS_ae_rl_r_dr_out/1
  FCS_ae_rl_r_dr/1 -> dr_l/1, RL2/1
  RL2/1 -> dr_actuator (with initial state)/1, dr_r/1

== system admire_sim_NDI/FCS_ae_rl/FCS_ae_rl_rc ==
  note: Level V
  FCS_ae_rl_rc_drc : Inport
  RL2 : RateLimiter  RisingSlewLimit=rlimit_c+ddc_rate  FallingSlewLimit=-rlimit_c-ddc_rate
  drc_actuator (with initial state) : simulink_extras/Additional Linear/Transfer Fcn (with initial states)  N=[1]  D="[0.05+ddc_bw  1]"  X0=x0(1)
  drc_l : ToWorkspace  VariableName=drc_l
  drc_r : ToWorkspace  VariableName=drc_r
  FCS_ae_rl_rc_drc_out : Outport  InitialOutput=0
  wires:
  drc_actuator (with initial state)/1 -> FCS_ae_rl_rc_drc_out/1
  FCS_ae_rl_rc_drc/1 -> drc_l/1, RL2/1
  RL2/1 -> drc_actuator (with initial state)/1, drc_r/1

== system admire_sim_NDI/FCS_ae_rl/FCS_ae_rl_rie ==
  note: Level V
  FCS_ae_rl_rie_drie : Inport
  RL2 : RateLimiter  RisingSlewLimit=rlimit_ie+ddei_rate  FallingSlewLimit=-rlimit_ie-ddei_rate
  drie_actuator (with initial state) : simulink_extras/Additional Linear/Transfer Fcn (with initial states)  N=[1]  D="[0.05+ddei_bw  1]"  X0=x0(4)
  drie_l : ToWorkspace  VariableName=drie_l
  drie_r : ToWorkspace  VariableName=drie_r
  FCS_ae_rl_rie_drie_out : Outport  InitialOutput=0
  wires:
  FCS_ae_rl_rie_drie/1 -> drie_l/1, RL2/1
  drie_actuator (with initial state)/1 -> FCS_ae_rl_rie_drie_out/1
  RL2/1 -> drie_r/1, drie_actuator (with initial state)/1

== system admire_sim_NDI/FCS_ae_rl/FCS_ae_rl_roe ==
  note: Level V
  FCS_ae_rl_roe_droe : Inport
  RL2 : RateLimiter  RisingSlewLimit=rlimit_oe+ddey_rate  FallingSlewLimit=-rlimit_oe-ddey_rate
  droe_actuator (with initial state) : simulink_extras/Additional Linear/Transfer Fcn (with initial states)  N=[1]  D="[0.05+ddey_bw  1]"  X0=x0(3)
  droe_l : ToWorkspace  VariableName=droe_l
  droe_r : ToWorkspace  VariableName=droe_r
  FCS_ae_rl_roe_droe_out : Outport  InitialOutput=0
  wires:
  droe_actuator (with initial state)/1 -> FCS_ae_rl_roe_droe_out/1
  FCS_ae_rl_roe_droe/1 -> droe_l/1, RL2/1
  RL2/1 -> droe_actuator (with initial state)/1, droe_r/1

== system admire_sim_NDI/NDI_CLAW/DynamicInversionControl ==
  INPUT : Inport
  MM : Inport  Port=2
  AERO_OBM : Subsystem
  Auto_Throttle : Subsystem
  Bus Selector : BusSelector  OutputSignals=CVdt_nom
  CMD : Subsystem
  ControlAllocation : Subsystem
  REG : Subsystem
  Scope : Scope  NumInputPorts=2
  Sum1 : Sum  Inputs=|+-
  To Workspace : ToWorkspace  VariableName=CVdt_des  SampleTime=-1
  To Workspace1 : ToWorkspace  VariableName=Ucmd  SampleTime=-1
  UcmdScope : Subsystem
  Unom : Subsystem
  DI_Cmds : Outport
  wires:
  INPUT/1 -> AERO_OBM/1(INPUT), Auto_Throttle/1(INPUT), REG/2(INPUT), CMD/2(INPUT)
  REG/1(CVdt_des) -> Sum1/1
  Sum1/1 -> Scope/1, ControlAllocation/3(CVdt_des), To Workspace/1  "dx_des-dx_nom"
  Auto_Throttle/1(TSS_cmd) -> ControlAllocation/1(TSS_cmd)
  ControlAllocation/1(Ucmd) -> DI_Cmds/1, To Workspace1/1, Unom/1(Ucmd), UcmdScope/1(In1)
  AERO_OBM/1(OBM) -> Bus Selector/1, ControlAllocation/4(OBM)
  Bus Selector/1 -> Sum1/2  "<CVdt_nom>"
  MM/1 -> CMD/1(MM)
  CMD/1(CMD) -> REG/1(CMD), Auto_Throttle/2(CMD)
  Auto_Throttle/2(UseSplit) -> ControlAllocation/2(UseSplit)
  Unom/1(Upast) -> AERO_OBM/2(uz)
  ControlAllocation/2(moment) -> Scope/2

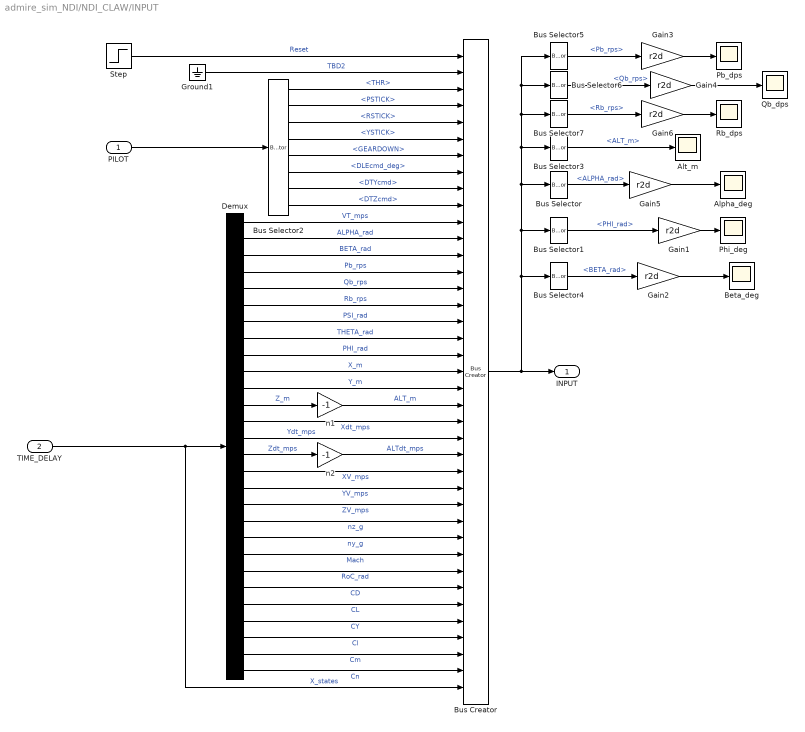
== system admire_sim_NDI/NDI_CLAW/INPUT ==
  PILOT : Inport
  TIME_DELAY : Inport  Port=2
  Alpha_deg : Scope
  Alt_m : Scope
  Beta_deg : Scope
  Bus Creator : BusCreator  Inputs=39
  Bus Selector : BusSelector  OutputSignals=ALPHA_rad
  Bus Selector1 : BusSelector  OutputSignals=PHI_rad
  Bus Selector2 : BusSelector  OutputSignals=THR,PSTICK,RSTICK,YSTICK,GEARDOWN,DLEcmd_deg,DTYcmd,DTZcmd
  Bus Selector3 : BusSelector  OutputSignals=ALT_m
  Bus Selector4 : BusSelector  OutputSignals=BETA_rad
  Bus Selector5 : BusSelector  OutputSignals=Pb_rps
  Bus Selector6 : BusSelector  OutputSignals=Qb_rps
  Bus Selector7 : BusSelector  OutputSignals=Rb_rps
  Demux : Demux  Outputs=28
  Gain{1..6} (6 alike) : Gain  Gain=r2d
  Ground1 : Ground
  Pb_dps : Scope
  Phi_deg : Scope
  Qb_dps : Scope
  Rb_dps : Scope
  Step : Step  Time=dt  Before=1  After=0  SampleTime=dt
  n1 : Gain  Gain=-1
  n2 : Gain  Gain=-1
  INPUT : Outport
  wires:
  Bus Creator/1 -> INPUT/1, Bus Selector3/1, Bus Selector5/1, Bus Selector6/1, Bus Selector7/1, Bus Selector/1, Bus Selector1/1, Bus Selector4/1
  PILOT/1 -> Bus Selector2/1
  Bus Selector2/1 -> Bus Creator/3  "<THR>"
  Bus Selector2/2 -> Bus Creator/4  "<PSTICK>"
  Bus Selector2/3 -> Bus Creator/5  "<RSTICK>"
  Bus Selector2/4 -> Bus Creator/6  "<YSTICK>"
  Bus Selector2/5 -> Bus Creator/7  "<GEARDOWN>"
  Ground1/1 -> Bus Creator/2  "TBD2"
  Step/1 -> Bus Creator/1  "Reset"
  Bus Selector2/6 -> Bus Creator/8  "<DLEcmd_deg>"
  Bus Selector2/7 -> Bus Creator/9  "<DTYcmd>"
  Bus Selector2/8 -> Bus Creator/10  "<DTZcmd>"
  Demux/1 -> Bus Creator/11  "VT_mps"
  Demux/2 -> Bus Creator/12  "ALPHA_rad"
  Demux/5 -> Bus Creator/15  "Qb_rps"
  Demux/8 -> Bus Creator/18  "THETA_rad"
  Demux/3 -> Bus Creator/13  "BETA_rad"
  Demux/4 -> Bus Creator/14  "Pb_rps"
  Demux/6 -> Bus Creator/16  "Rb_rps"
  Demux/9 -> Bus Creator/19  "PHI_rad"
  Demux/10 -> Bus Creator/20  "X_m"
  Demux/11 -> Bus Creator/21  "Y_m"
  Demux/12 -> n1/1  "Z_m"
  n1/1 -> Bus Creator/22  "ALT_m"
  Demux/13 -> Bus Creator/23  "Xdt_mps"
  Demux/14 -> Bus Creator/24  "Ydt_mps"
  Demux/15 -> n2/1  "Zdt_mps"
  Demux/16 -> Bus Creator/26  "XV_mps"
  Demux/17 -> Bus Creator/27  "YV_mps"
  Demux/18 -> Bus Creator/28  "ZV_mps"
  Demux/19 -> Bus Creator/29  "nz_g"
  Demux/20 -> Bus Creator/30  "ny_g"
  Demux/21 -> Bus Creator/31  "Mach"
  Demux/22 -> Bus Creator/32  "RoC_rad"
  Demux/23 -> Bus Creator/33  "CD"
  Demux/24 -> Bus Creator/34  "CL"
  Demux/25 -> Bus Creator/35  "CY"
  Demux/26 -> Bus Creator/36  "Cl"
  Demux/27 -> Bus Creator/37  "Cm"
  Demux/28 -> Bus Creator/38  "Cn"
  Demux/7 -> Bus Creator/17  "PSI_rad"
  n2/1 -> Bus Creator/25  "ALTdt_mps"
  TIME_DELAY/1 -> Demux/1, Bus Creator/39  "X_states"
  Gain5/1 -> Alpha_deg/1
  Bus Selector/1 -> Gain5/1  "<ALPHA_rad>"
  Gain1/1 -> Phi_deg/1
  Bus Selector1/1 -> Gain1/1  "<PHI_rad>"
  Bus Selector3/1 -> Alt_m/1  "<ALT_m>"
  Gain2/1 -> Beta_deg/1
  Bus Selector4/1 -> Gain2/1  "<BETA_rad>"
  Bus Selector5/1 -> Gain3/1  "<Pb_rps>"
  Bus Selector6/1 -> Gain4/1  "<Qb_rps>"
  Bus Selector7/1 -> Gain6/1  "<Rb_rps>"
  Gain3/1 -> Pb_dps/1
  Gain4/1 -> Qb_dps/1
  Gain6/1 -> Rb_dps/1

== system admire_sim_NDI/NDI_CLAW/MissionManager ==
  INPUT : Inport
  ALT_table : Lookup  InputValues=Altcmd_t  Table=Altcmd_v  LookUpMeth=Interpolation-Use End Values
  Bus Creator : BusCreator  Inputs=8
  Bus Selector3 : BusSelector  OutputSignals=Xcmd,Xcmdm1,Ycmd,Ycmdm1,PHImax_rad
  Constant : Constant  Value=Vcmd_v(1)
  Constant1 : Constant  Value=Altcmd_v(1)
  Constant2 : Constant  Value=x0bare(1)
  Constant3 : Constant  Value=-x0bare(12)+50
  Constant4 : Constant  Value=-120
  Digital Clock : DigitalClock  SampleTime=dt
  Gain : Gain  Gain=0
  PHI_5 : Lookup  InputValues=PHIcmd_t  Table=PHIcmd_v  LookUpMeth=Interpolation-Use End Values
  Saturation : Saturate  UpperLimit=300  LowerLimit=0
  Sum : Sum  Inputs=|++
  V_table : Lookup  InputValues=Vcmd_t  Table=Vcmd_v  LookUpMeth=Interpolation-Use End Values
  WaypointNavigation : Subsystem
  MM : Outport
  wires:
  Digital Clock/1 -> Sum/1, V_table/1, ALT_table/1
  Bus Creator/1 -> MM/1
  PHI_5/1 -> Bus Creator/3  "PHIcmd_deg"
  INPUT/1 -> WaypointNavigation/1(INPUT)
  WaypointNavigation/1(WN) -> Bus Selector3/1
  Bus Selector3/1 -> Bus Creator/4  "<Xcmd>"
  Bus Selector3/2 -> Bus Creator/5  "<Xcmdm1>"
  Bus Selector3/3 -> Bus Creator/6  "<Ycmd>"
  Bus Selector3/4 -> Bus Creator/7  "<Ycmdm1>"
  Bus Selector3/5 -> Bus Creator/8  "<PHImax_rad>"
  V_table/1 -> Bus Creator/2  "Vcmd_mps"
  ALT_table/1 -> Bus Creator/1  "ALTcmd_m"
  Sum/1 -> Saturation/1
  Constant4/1 -> Sum/2
  Saturation/1 -> Gain/1
  Gain/1 -> PHI_5/1

== system admire_sim_NDI/NDI_CLAW/PILOT_Mod ==
  In1 : Inport
  Bus Creator1 : BusCreator  Inputs=9
  Bus Selector : BusSelector  OutputSignals=Fes_out,Vt_out,Fas_out,Frp_out,dle_out,ldg_out,dty_out,dtz_out,tss_out
  Gain1 : Gain  Gain=1/80
  Gain{2,5..9} (6 alike) : Gain
  Gain3 : Gain  Gain=1/80
  Gain4 : Gain  Gain=1/200
  PILOT : Outport
  wires:
  In1/1 -> Bus Selector/1
  Bus Selector/1 -> Gain1/1  "<Fes_out>"
  Bus Selector/2 -> Gain2/1  "<Vt_out>"
  Bus Selector/3 -> Gain3/1  "<Fas_out>"
  Bus Selector/4 -> Gain4/1  "<Frp_out>"
  Bus Selector/5 -> Gain5/1  "<dle_out>"
  Bus Selector/6 -> Gain6/1  "<ldg_out>"
  Bus Selector/7 -> Gain7/1  "<dty_out>"
  Bus Selector/8 -> Gain8/1  "<dtz_out>"
  Gain1/1 -> Bus Creator1/1  "PSTICK"
  Gain2/1 -> Bus Creator1/2  "Vcmd_mps"
  Gain3/1 -> Bus Creator1/3  "RSTICK"
  Gain4/1 -> Bus Creator1/4  "YSTICK"
  Gain5/1 -> Bus Creator1/5  "DLEcmd_deg"
  Gain6/1 -> Bus Creator1/6  "GEARDOWN"
  Gain7/1 -> Bus Creator1/7  "DTYcmd"
  Gain8/1 -> Bus Creator1/8  "DTZcmd"
  Gain9/1 -> Bus Creator1/9  "THR"
  Bus Creator1/1 -> PILOT/1
  Bus Selector/9 -> Gain9/1  "<tss_out>"

== system admire_sim_NDI/PILOT/Doublet ==
  Gain : Gain  Gain=.1
  Step : Step  SampleTime=0
  Step1 : Step  Time=1.1  After=-2  SampleTime=0
  Step2 : Step  Time=1.2  SampleTime=0
  Sum8 : Sum  Inputs=+++
  Out1 : Outport
  wires:
  Step/1 -> Sum8/1
  Step1/1 -> Sum8/2
  Step2/1 -> Sum8/3
  Sum8/1 -> Gain/1
  Gain/1 -> Out1/1

== system admire_sim_NDI/Aircraft response1/Sensor models/Subsystem To Gain-Scheduling ==
  note: Level III
  Vt [m/s] : Inport
  alt [m] : Inport  Port=2
  S-Function : S-Function  FunctionName=machno  SFunctionDeploymentMode=off  EnableBusSupport=off
  Mach : Outport
  tag scope: Altitude=global, Mach=global
  wires:
  alt [m]/1 -> [Altitude], S-Function/2
  Vt [m/s]/1 -> S-Function/1
  S-Function/1 -> [Mach], Mach/1
